simulink model "Mdl_Dim"  (R2024b)
settings: Solver=FixedStepDiscrete  StartTime=0.0  StopTime=10.0  FixedStep=0.1  RelTol=1e-3  EnableMultiTasking=on
values from neighbouring files (symbols this model uses):
  DEFAULT_MODE = mpt.Parameter    [Mdl_Dim_DD.m]
  DEFAULT_STEP = mpt.Parameter    [Mdl_Dim_DD.m]
  Mdl_Dim_cTaskPeriod = mpt.Parameter    [Mdl_Dim_rte_types.m]
  RTE_E_MAX_AGE_EXCEEDED = mpt.Parameter    [Mdl_Dim_rte_types.m]
  RTE_E_NEVER_RECEIVED = mpt.Parameter    [Mdl_Dim_rte_types.m]
  STATUS_OFF = mpt.Parameter    [Mdl_Dim_DD.m]
  STATUS_ON = mpt.Parameter    [Mdl_Dim_DD.m]
  SWITCHING_MECHANISM = mpt.Parameter    [Mdl_Dim_DD.m]
  ZERO_VAL = mpt.Parameter    [Mdl_Dim_DD.m]
undefined symbols (not defined in the file or in its folder): AppModule, CAN_COMUN_ACTIVE, CAN_COMUN_FAIL, CAN_VAL_OFF, CAN_VAL_ON, ChannelID, CLUSTER_ACTIVE, DAYNIGHT_STS_NOTRequire, DIAG_NCTRL, DIM_DAY_MODE, DIM_NIGHT_MODE, DOWN_THRESH_1SW, DrvRec_Rheo_down_Long_Press, DrvRec_Rheo_down_Short_Press, DrvRec_Rheo_up_Long_Press, DrvRec_Rheo_Up_Short_Press, DW_EVENT, DW_ON, eAppMdl_type_instance, eDayNightModeIn, eIllumination_levelIn, eSIGNAL_MISSING, eSIGNAL_NEVER_RECEIVED, eSleepSt_type_instance, FALSE, GetPwmDirect, GetPwmWithTime, GetPwmWithTimeExp, IgnOn, INDEX_MCUID0340, INDEX_MCUID0341, INDEX_MCUID0430, IoHwAb_PwmSignalIdType_type_instance, l_Wheel_Down_ParamArray, l_Wheel_Up_ParamArray, MAX_UINT16, MAXHOLD, MINHOLD, NETWORK_NORMAL, NETWORK_SLEEP, NETWORK_STANDALONE, NONE, NVM_Adapter_SetNVM_RheostatDayStep, NVM_Adapter_SetNVM_RheostatDayStepU1, NVM_Adapter_SetNVM_RheostatDayStepU2, NVM_Adapter_SetNVM_RheostatDayStepU3, NVM_Adapter_SetNVM_RheostatNightStep, NVM_Adapter_SetNVM_RheostatNightStepU1, NVM_Adapter_SetNVM_RheostatNightStepU2, NVM_Adapter_SetNVM_RheostatNightStepU3, OpeModeRheostatChange, pJustRcvdStatus, pNvmData, POS_MAX, POS_MIN, RHEO_1SW_TYPE, RHEO_2SW_TYPE, RHEO_SOFTSW_TYPE, RHEO_VALUE_FIVE_U16, RHEO_VALUE_ONE_BOOL ... (+48)
libraries: simulink x65
(part 1 of 4)
settings Model: Creator=AELANGO6  LastModifiedBy=AELANGO6
settings DataIOCC: SaveOutput=off
settings OptimizationCC: DefaultParameterBehavior=Inlined  EnhancedBackFolding=on  PassReuseOutputArgsAs=Individual arguments  ZeroExternalMemoryAtStartup=off  ZeroInternalMemoryAtStartup=off  MaxStackSize=750  OptimizeBlockOrder=speed  DifferentSizesBufferReuse=on  OptimizationCustomize=off  EfficientTunableParamExpr=on
settings DebuggingCC: ParameterTunabilityLossMsg=error
settings SFSimCC: MATLABDynamicMemAlloc=off
settings RTWCC: Description=AUTOSAR  SystemTargetFile=autosar.tlc  GenCodeOnly=on  TemplateMakefile=ert_default_tmf  PortableWordSizes=on  DataTypeReplacement=CDataTypesFixedWidth
settings CodeAppCC: ForceParamTrailComments=on  IgnoreCustomStorageClasses=off  OperatorAnnotations=on  SimulinkDataObjDesc=on  SFDataObjDesc=on  InsertBlockDesc=on
settings STFCustomTargetCC: TargetLangStandard=C99 (ISO)  MultiwordLength=256  ParMdlRefBuildCompliant=on  CompOptLevelCompliant=on  IncludeMdlTerminateFcn=off  CombineOutputUpdateFcns=on  SuppressErrorStatus=on  ERTCustomFileBanners=on  SupportNonFinite=off  SupportComplex=off  SupportContinuousTime=off  SupportNonInlinedSFcns=off  RemoveResetFunc=on  ParenthesesLevel=Maximum  CastingMode=Standards  MATLABClassNameForMDSCustomization=Simulink.SoftwareTarget.ERTCustomization  AutosarCompliant=on  UseToolchainInfoCompliant=on  LookupTableObjectStructAxisOrder=2,1,3,4,...  LUTObjectStructOrderEvenSpacing=Size,Table,Breakpoints  SystemTargetFile=autosar.tlc
settings ERTTargetCC: TargetLangStandard=C99 (ISO)  ConcurrentExecutionCompliant=off  IncludeMdlTerminateFcn=off  SuppressErrorStatus=on  SupportNonFinite=off  SupportComplex=off  ParenthesesLevel=Maximum  CastingMode=Standards  ModelStepFunctionPrototypeControlCompliant=off  CPPClassGenCompliant=off  AutosarCompliant=on  LookupTableObjectStructAxisOrder=2,1,3,4,...  LUTObjectStructOrderEvenSpacing=Size,Table,Breakpoints  ERTCustomFileTemplate=example_file_process.tlc  ERTFilePackagingFormat=CompactWithDataFile  BooleanTrueId=TRUE  BooleanFalseId=FALSE

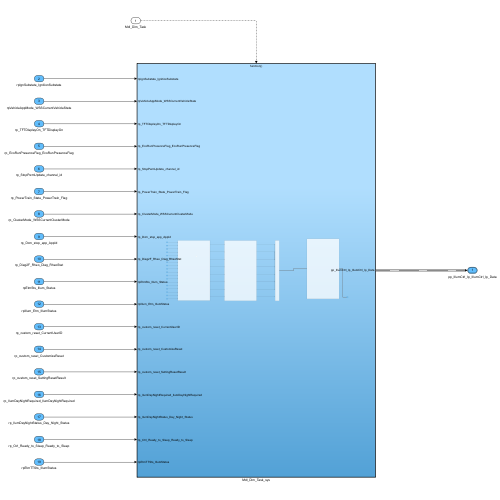
[thumbnail: Simulink's stored preview of the top-level diagram]
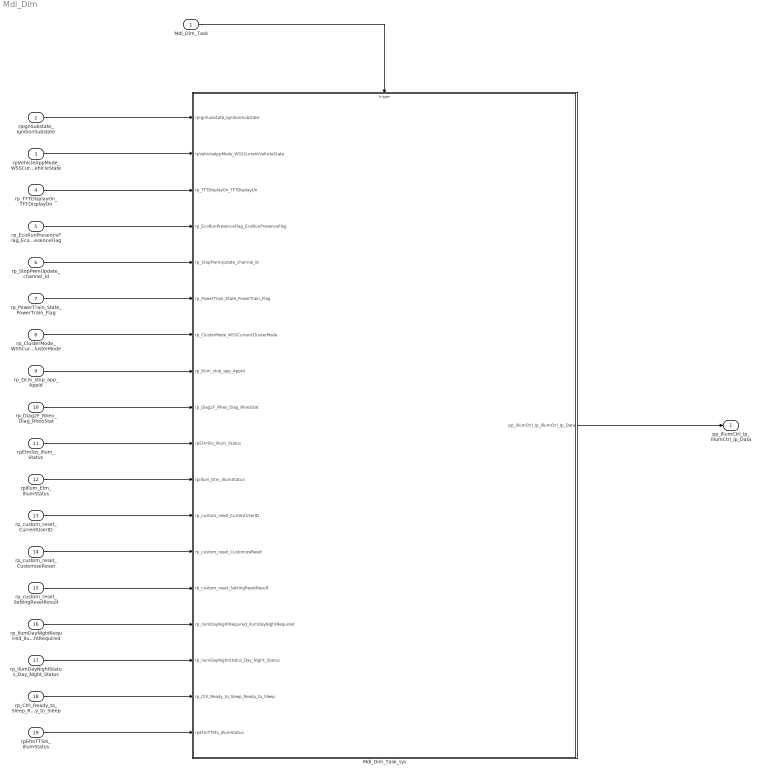
== system Mdl_Dim ==
  Mdl_Dim_Task : Inport  SampleTime=0.1  OutputFunctionCall=on
  rpIgnSubstate_IgnitionSubstate : Inport  Port=2  OutDataTypeStr=IgntionSubstateType  PortDimensions=1
  rpVehicleAppMode_WSSCurrentVehicleState : Inport  Port=3  OutDataTypeStr=VehicleActiveModes  PortDimensions=1
  rp_TFTDisplayOn_TFTDisplayOn : Inport  Port=4  OutDataTypeStr=DisplayStatus  PortDimensions=1
  rp_EcoRunPresenceFlag_EcoRunPresenceFlag : Inport  Port=5  OutDataTypeStr=uint8  PortDimensions=1
  rp_StopPwmUpdate_channel_id : Inport  Port=6  OutDataTypeStr=uint8  PortDimensions=1
  rp_PowerTrain_State_PowerTrain_Flag : Inport  Port=7  OutDataTypeStr=uint8  PortDimensions=1
  rp_ClusterMode_WSSCurrentClusterMode : Inport  Port=8  OutDataTypeStr=ClusterModes  PortDimensions=1
  rp_Dcm_stop_app_AppId : Inport  Port=9  OutDataTypeStr=IOCtrl_Type  PortDimensions=1
  rp_Diag2F_Rheo_Diag_RheoStat : Inport  Port=10  OutDataTypeStr=uint8  PortDimensions=1
  rpEtmSts_Illum_Status : Inport  Port=11  OutDataTypeStr=uint8  PortDimensions=1
  rpIllum_Etm_IllumStatus : Inport  Port=12  OutDataTypeStr=uint8  PortDimensions=1
  rp_custom_reset_CurrentUserID : Inport  Port=13  OutDataTypeStr=UserIdType  PortDimensions=1
  rp_custom_reset_CustomizeReset : Inport  Port=14  OutDataTypeStr=CustResetType  PortDimensions=1
  rp_custom_reset_SettingResetResult : Inport  Port=15  OutDataTypeStr=SettingResetResult_Type  PortDimensions=1
  rp_IlumDayNightRequired_IlumDayNightRequired : Inport  Port=16  OutDataTypeStr=uint8  PortDimensions=1
  rp_IlumDayNightStatus_Day_Night_Status : Inport  Port=17  OutDataTypeStr=uint8  PortDimensions=1
  rp_Ctrl_Ready_to_Sleep_Ready_to_Sleep : Inport  Port=18  OutDataTypeStr=boolean  PortDimensions=1
  rpEtmTTSts_IllumStatus : Inport  Port=19  OutDataTypeStr=uint8  PortDimensions=1
  Mdl_Dim_Task_sys : Subsystem  TreatAsAtomicUnit=on
  pp_IllumCtrl_Ip_IllumCtrl_Ip_Data : Outport  OutDataTypeStr=Bus:IllumCtrl_Ip
  wires:
  Mdl_Dim_Task/1 -> Mdl_Dim_Task_sys/Trigger
  rp_PowerTrain_State_PowerTrain_Flag/1 -> Mdl_Dim_Task_sys/6(rp_PowerTrain_State_PowerTrain_Flag)
  rpIgnSubstate_IgnitionSubstate/1 -> Mdl_Dim_Task_sys/1(rpIgnSubstate_IgnitionSubstate)
  rp_custom_reset_CurrentUserID/1 -> Mdl_Dim_Task_sys/12(rp_custom_reset_CurrentUserID)
  rpVehicleAppMode_WSSCurrentVehicleState/1 -> Mdl_Dim_Task_sys/2(rpVehicleAppMode_WSSCurrentVehicleState)
  rp_TFTDisplayOn_TFTDisplayOn/1 -> Mdl_Dim_Task_sys/3(rp_TFTDisplayOn_TFTDisplayOn)
  rp_IlumDayNightStatus_Day_Night_Status/1 -> Mdl_Dim_Task_sys/16(rp_IlumDayNightStatus_Day_Night_Status)
  rp_EcoRunPresenceFlag_EcoRunPresenceFlag/1 -> Mdl_Dim_Task_sys/4(rp_EcoRunPresenceFlag_EcoRunPresenceFlag)
  rp_StopPwmUpdate_channel_id/1 -> Mdl_Dim_Task_sys/5(rp_StopPwmUpdate_channel_id)
  rp_ClusterMode_WSSCurrentClusterMode/1 -> Mdl_Dim_Task_sys/7(rp_ClusterMode_WSSCurrentClusterMode)
  rp_Dcm_stop_app_AppId/1 -> Mdl_Dim_Task_sys/8(rp_Dcm_stop_app_AppId)
  rp_Diag2F_Rheo_Diag_RheoStat/1 -> Mdl_Dim_Task_sys/9(rp_Diag2F_Rheo_Diag_RheoStat)
  rpEtmSts_Illum_Status/1 -> Mdl_Dim_Task_sys/10(rpEtmSts_Illum_Status)
  rpIllum_Etm_IllumStatus/1 -> Mdl_Dim_Task_sys/11(rpIllum_Etm_IllumStatus)
  rp_custom_reset_CustomizeReset/1 -> Mdl_Dim_Task_sys/13(rp_custom_reset_CustomizeReset)
  rp_custom_reset_SettingResetResult/1 -> Mdl_Dim_Task_sys/14(rp_custom_reset_SettingResetResult)
  rp_IlumDayNightRequired_IlumDayNightRequired/1 -> Mdl_Dim_Task_sys/15(rp_IlumDayNightRequired_IlumDayNightRequired)
  rp_Ctrl_Ready_to_Sleep_Ready_to_Sleep/1 -> Mdl_Dim_Task_sys/17(rp_Ctrl_Ready_to_Sleep_Ready_to_Sleep)
  Mdl_Dim_Task_sys/1(pp_IllumCtrl_Ip_IllumCtrl_Ip_Data) -> pp_IllumCtrl_Ip_IllumCtrl_Ip_Data/1
  rpEtmTTSts_IllumStatus/1 -> Mdl_Dim_Task_sys/18(rpEtmTTSts_IllumStatus)

== system Mdl_Dim/Mdl_Dim_Task_sys ==
  rpIgnSubstate_IgnitionSubstate : Inport  OutDataTypeStr=IgntionSubstateType  PortDimensions=1
  rpVehicleAppMode_WSSCurrentVehicleState : Inport  Port=2  OutDataTypeStr=VehicleActiveModes  PortDimensions=1
  rp_TFTDisplayOn_TFTDisplayOn : Inport  Port=3  OutDataTypeStr=DisplayStatus  PortDimensions=1
  rp_EcoRunPresenceFlag_EcoRunPresenceFlag : Inport  Port=4  OutDataTypeStr=uint8  PortDimensions=1
  rp_StopPwmUpdate_channel_id : Inport  Port=5  OutDataTypeStr=uint8  PortDimensions=1
  rp_PowerTrain_State_PowerTrain_Flag : Inport  Port=6  OutDataTypeStr=uint8  PortDimensions=1
  rp_ClusterMode_WSSCurrentClusterMode : Inport  Port=7  OutDataTypeStr=ClusterModes  PortDimensions=1
  rp_Dcm_stop_app_AppId : Inport  Port=8  OutDataTypeStr=IOCtrl_Type  PortDimensions=1
  rp_Diag2F_Rheo_Diag_RheoStat : Inport  Port=9  OutDataTypeStr=uint8  PortDimensions=1
  rpEtmSts_Illum_Status : Inport  Port=10  OutDataTypeStr=uint8  PortDimensions=1
  rpIllum_Etm_IllumStatus : Inport  Port=11  OutDataTypeStr=uint8  PortDimensions=1
  rp_custom_reset_CurrentUserID : Inport  Port=12  OutDataTypeStr=UserIdType  PortDimensions=1
  rp_custom_reset_CustomizeReset : Inport  Port=13  OutDataTypeStr=CustResetType  PortDimensions=1
  rp_custom_reset_SettingResetResult : Inport  Port=14  OutDataTypeStr=SettingResetResult_Type  PortDimensions=1
  rp_IlumDayNightRequired_IlumDayNightRequired : Inport  Port=15  OutDataTypeStr=uint8  PortDimensions=1
  rp_IlumDayNightStatus_Day_Night_Status : Inport  Port=16  OutDataTypeStr=uint8  PortDimensions=1
  rp_Ctrl_Ready_to_Sleep_Ready_to_Sleep : Inport  Port=17  OutDataTypeStr=boolean  PortDimensions=1
  rpEtmTTSts_IllumStatus : Inport  Port=18  OutDataTypeStr=uint8  PortDimensions=1
  function : TriggerPort  TriggerType=function-call  VariantControl=(inherit)  SampleTimeType=periodic  SampleTime=-1
  IllumCtrl_Ip_Data_creator : BusCreator  Inputs=8  OutDataTypeStr=Bus:IllumCtrl_Ip  NonVirtualBus=on
  InputHarness : Subsystem  Variant=on
  OutputHarness : Subsystem  Variant=on
  Subsystem : Subsystem
  pp_IllumCtrl_Ip_IllumCtrl_Ip_Data : Outport  OutDataTypeStr=Bus:IllumCtrl_Ip  PortDimensions=1
  wires:
  rpIgnSubstate_IgnitionSubstate/1 -> InputHarness/1(rpIgnSubstate_IgnitionSubstate)
  rpVehicleAppMode_WSSCurrentVehicleState/1 -> InputHarness/2(rpVehicleAppMode_WSSCurrentVehicleState)
  rp_TFTDisplayOn_TFTDisplayOn/1 -> InputHarness/3(rp_TFTDisplayOn_TFTDisplayOn)
  rp_EcoRunPresenceFlag_EcoRunPresenceFlag/1 -> InputHarness/4(rp_EcoRunPresenceFlag_EcoRunPresenceFlag)
  rp_StopPwmUpdate_channel_id/1 -> InputHarness/5(rp_StopPwmUpdate_channel_id)
  rp_PowerTrain_State_PowerTrain_Flag/1 -> InputHarness/6(rp_PowerTrain_State_PowerTrain_Flag)
  rp_ClusterMode_WSSCurrentClusterMode/1 -> InputHarness/7(rp_ClusterMode_WSSCurrentClusterMode)
  rp_Dcm_stop_app_AppId/1 -> InputHarness/8(rp_Dcm_stop_app_AppId)
  rp_Diag2F_Rheo_Diag_RheoStat/1 -> InputHarness/9(rp_Diag2F_Rheo_Diag_RheoStat)
  rpEtmSts_Illum_Status/1 -> InputHarness/10(rpEtmSts_Illum_Status)
  rpIllum_Etm_IllumStatus/1 -> InputHarness/11(rpIllum_Etm_IllumStatus)
  rp_custom_reset_CurrentUserID/1 -> InputHarness/12(rp_custom_reset_CurrentUserID)
  rp_custom_reset_CustomizeReset/1 -> InputHarness/13(rp_custom_reset_CustomizeReset)
  rp_custom_reset_SettingResetResult/1 -> InputHarness/14(rp_custom_reset_SettingResetResult)
  rp_IlumDayNightRequired_IlumDayNightRequired/1 -> InputHarness/15(rp_IlumDayNightRequired_IlumDayNightRequired)
  rp_IlumDayNightStatus_Day_Night_Status/1 -> InputHarness/16(rp_IlumDayNightStatus_Day_Night_Status)
  rp_Ctrl_Ready_to_Sleep_Ready_to_Sleep/1 -> InputHarness/17(rp_Ctrl_Ready_to_Sleep_Ready_to_Sleep)
  rpEtmTTSts_IllumStatus/1 -> InputHarness/18(rpEtmTTSts_IllumStatus)
  InputHarness/1(rpIgnSubstate_IgnitionSubstate_out) -> Subsystem/1(IgnitionSubstate)
  InputHarness/2(rpVehicleAppMode_WSSCurrentVehicleState_out) -> Subsystem/2(VehicleState)
  InputHarness/3(rp_TFTDisplayOn_TFTDisplayOn_out) -> Subsystem/3(TFTDisplayOn)
  InputHarness/4(rp_ClusterMode_WSSCurrentClusterMode_out) -> Subsystem/4(cluster_Active_check)
  OutputHarness/1(pp_IllumCtrl_Ip_IllumCtrl_Ip_Data) -> pp_IllumCtrl_Ip_IllumCtrl_Ip_Data/1
  IllumCtrl_Ip_Data_creator/1 -> OutputHarness/1(pp_IllumCtrl_Ip_IllumCtrl_Ip_Data_in)  "fl_IllumMdl_Op"
  InputHarness/5(IL_Mode_CAN_Data) -> Subsystem/5(IL_Mode_Can_Data)
  InputHarness/6(IL_Mode_CAN_Status) -> Subsystem/6(IL_Mode_Can_Sts)
  InputHarness/7(IL_Level_CAN_Data) -> Subsystem/7(IL_Level_Can_Data)
  InputHarness/8(IL_Level_CAN_Status) -> Subsystem/8(IL_Level_Can_Sts)
  Subsystem/1(power_mode) -> IllumCtrl_Ip_Data_creator/4  "power_mode"
  Subsystem/2(Illumination_Sts) -> IllumCtrl_Ip_Data_creator/3  "Illumination_Sts"
  Subsystem/3(Illumination_Mode) -> IllumCtrl_Ip_Data_creator/1  "Illumination_Mode"
  Subsystem/4(step_value) -> IllumCtrl_Ip_Data_creator/5  "step_value"
  Subsystem/5(switch_type) -> IllumCtrl_Ip_Data_creator/7  "switch_type"
  Subsystem/6(battery_status) -> IllumCtrl_Ip_Data_creator/2  "battery_status"
  Subsystem/7(step_direction) -> IllumCtrl_Ip_Data_creator/6  "step_direction"
  Subsystem/8(derating_value) -> IllumCtrl_Ip_Data_creator/8  "Derating_Value"

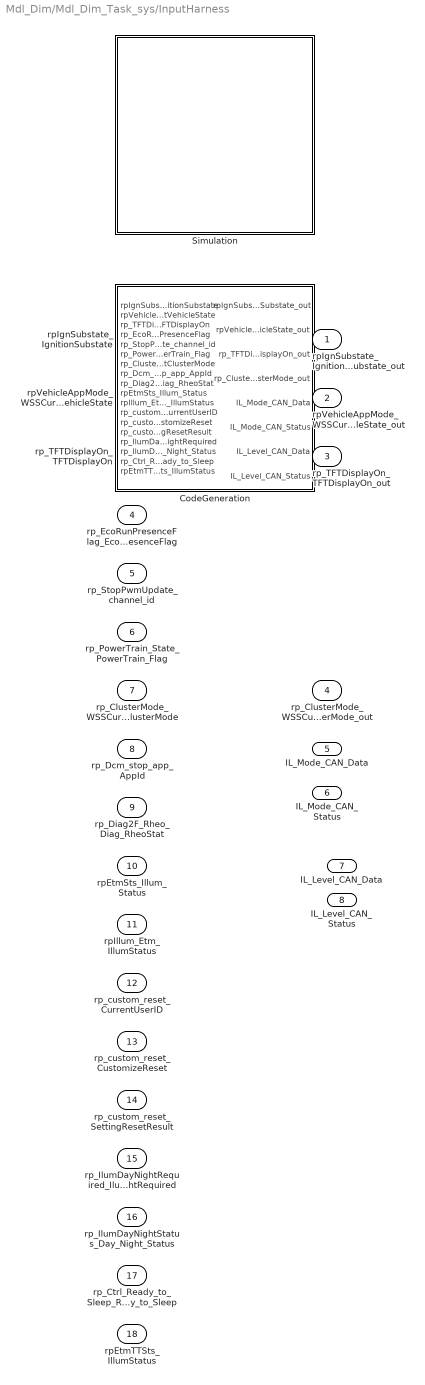
== system Mdl_Dim/Mdl_Dim_Task_sys/InputHarness ==
  rpIgnSubstate_IgnitionSubstate : Inport  OutDataTypeStr=IgntionSubstateType  PortDimensions=1
  rpVehicleAppMode_WSSCurrentVehicleState : Inport  Port=2  OutDataTypeStr=VehicleActiveModes  PortDimensions=1
  rp_TFTDisplayOn_TFTDisplayOn : Inport  Port=3  OutDataTypeStr=DisplayStatus  PortDimensions=1
  rp_EcoRunPresenceFlag_EcoRunPresenceFlag : Inport  Port=4  OutDataTypeStr=uint8  PortDimensions=1
  rp_StopPwmUpdate_channel_id : Inport  Port=5  OutDataTypeStr=uint8  PortDimensions=1
  rp_PowerTrain_State_PowerTrain_Flag : Inport  Port=6  OutDataTypeStr=uint8  PortDimensions=1
  rp_ClusterMode_WSSCurrentClusterMode : Inport  Port=7  OutDataTypeStr=ClusterModes  PortDimensions=1
  rp_Dcm_stop_app_AppId : Inport  Port=8  OutDataTypeStr=IOCtrl_Type  PortDimensions=1
  rp_Diag2F_Rheo_Diag_RheoStat : Inport  Port=9  OutDataTypeStr=uint8  PortDimensions=1
  rpEtmSts_Illum_Status : Inport  Port=10  OutDataTypeStr=uint8  PortDimensions=1
  rpIllum_Etm_IllumStatus : Inport  Port=11  OutDataTypeStr=uint8  PortDimensions=1
  rp_custom_reset_CurrentUserID : Inport  Port=12  OutDataTypeStr=UserIdType  PortDimensions=1
  rp_custom_reset_CustomizeReset : Inport  Port=13  OutDataTypeStr=CustResetType  PortDimensions=1
  rp_custom_reset_SettingResetResult : Inport  Port=14  OutDataTypeStr=SettingResetResult_Type  PortDimensions=1
  rp_IlumDayNightRequired_IlumDayNightRequired : Inport  Port=15  OutDataTypeStr=uint8  PortDimensions=1
  rp_IlumDayNightStatus_Day_Night_Status : Inport  Port=16  OutDataTypeStr=uint8  PortDimensions=1
  rp_Ctrl_Ready_to_Sleep_Ready_to_Sleep : Inport  Port=17  OutDataTypeStr=boolean  PortDimensions=1
  rpEtmTTSts_IllumStatus : Inport  Port=18  OutDataTypeStr=uint8  PortDimensions=1
  CodeGeneration : Subsystem  VariantControl=CODEGENERATION
  Simulation : Subsystem  VariantControl=SIMULATION
  rpIgnSubstate_IgnitionSubstate_out : Outport  OutDataTypeStr=IgntionSubstateType  PortDimensions=1
  rpVehicleAppMode_WSSCurrentVehicleState_out : Outport  Port=2  OutDataTypeStr=VehicleActiveModes  PortDimensions=1
  rp_TFTDisplayOn_TFTDisplayOn_out : Outport  Port=3  OutDataTypeStr=DisplayStatus  PortDimensions=1
  rp_ClusterMode_WSSCurrentClusterMode_out : Outport  Port=4  OutDataTypeStr=ClusterModes  PortDimensions=1
  IL_Mode_CAN_Data : Outport  Port=5
  IL_Mode_CAN_Status : Outport  Port=6
  IL_Level_CAN_Data : Outport  Port=7
  IL_Level_CAN_Status : Outport  Port=8

== system Mdl_Dim/Mdl_Dim_Task_sys/OutputHarness ==
  pp_IllumCtrl_Ip_IllumCtrl_Ip_Data_in : Inport  OutDataTypeStr=Bus:IllumCtrl_Ip  PortDimensions=1
  CodeGeneration : Subsystem  VariantControl=CODEGENERATION
  Simulation : Subsystem  VariantControl=SIMULATION
  pp_IllumCtrl_Ip_IllumCtrl_Ip_Data : Outport  OutDataTypeStr=Bus:IllumCtrl_Ip  PortDimensions=1

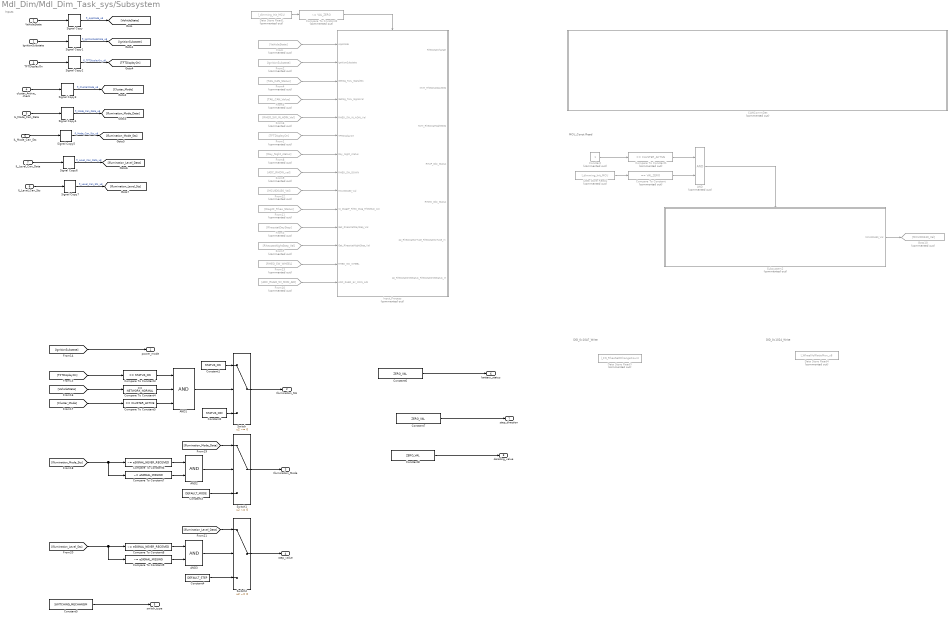
== system Mdl_Dim/Mdl_Dim_Task_sys/Subsystem ==
  note: Inputs
  note: MCU_Const Read
  note: DID_0x10A7_Write
  note: DID_0x1024_Write
  IgnitionSubstate : Inport
  VehicleState : Inport  Port=2
  TFTDisplayOn : Inport  Port=3
  cluster_Active_check : Inport  Port=4
  IL_Mode_Can_Data : Inport  Port=5
  IL_Mode_Can_Sts : Inport  Port=6
  IL_Level_Can_Data : Inport  Port=7
  IL_Level_Can_Sts : Inport  Port=8
  AND : Logic  Commented=on  AllPortsSameDT=off  OutDataTypeStr=boolean
  AND1 : Logic  Inputs=3  AllPortsSameDT=off  OutDataTypeStr=boolean
  AND2 : Logic  AllPortsSameDT=off  OutDataTypeStr=boolean
  AND3 : Logic  AllPortsSameDT=off  OutDataTypeStr=boolean
  CANCommDet : Subsystem  Commented=on  TreatAsAtomicUnit=on
  Compare To Constant : simulink/Logic and Bit Operations/Compare To Constant  Commented=on  relop===  const=VAL_ZERO  OutDataTypeStr=boolean
  Compare To Constant1 : simulink/Logic and Bit Operations/Compare To Constant  Commented=on  relop===  const=CLUSTER_ACTIVE  OutDataTypeStr=boolean
  Compare To Constant2 : simulink/Logic and Bit Operations/Compare To Constant  Commented=on  relop=~=  const=VAL_ZERO  OutDataTypeStr=boolean
  Compare To Constant3 : simulink/Logic and Bit Operations/Compare To Constant  relop===  const=STATUS_ON  OutDataTypeStr=boolean
  Compare To Constant4 : simulink/Logic and Bit Operations/Compare To Constant  relop===  const=NETWORK_NORMAL  OutDataTypeStr=boolean
  Compare To Constant5 : simulink/Logic and Bit Operations/Compare To Constant  relop===  const=CLUSTER_ACTIVE  OutDataTypeStr=boolean
  Compare To Constant6 : simulink/Logic and Bit Operations/Compare To Constant  relop=~=  const=eSIGNAL_NEVER_RECEIVED  OutDataTypeStr=boolean
  Compare To Constant7 : simulink/Logic and Bit Operations/Compare To Constant  relop=~=  const=eSIGNAL_MISSING  OutDataTypeStr=boolean
  Compare To Constant8 : simulink/Logic and Bit Operations/Compare To Constant  relop=~=  const=eSIGNAL_NEVER_RECEIVED  OutDataTypeStr=boolean
  Compare To Constant9 : simulink/Logic and Bit Operations/Compare To Constant  relop=~=  const=eSIGNAL_MISSING  OutDataTypeStr=boolean
  Constant : Constant  Commented=on
  Constant1 : Constant  Value=STATUS_ON
  Constant2 : Constant  Value=STATUS_OFF
  Constant3 : Constant  Value=DEFAULT_MODE
  Constant4 : Constant  Value=DEFAULT_STEP
  Constant5 : Constant  Value=SWITCHING_MECHANISM
  Constant6 : Constant  Value=ZERO_VAL
  Constant7 : Constant  Value=ZERO_VAL
  Constant8 : Constant  Value=ZERO_VAL
  Data Store Read1 : DataStoreRead  Commented=on  DataStoreName=l_dimming_Init_MCU  IndexOptions=Index vector (dialog)  Indices=1  OutputSizes=1
  Data Store Read2 : DataStoreRead  Commented=on  DataStoreName=l_dimming_Init_MCU  IndexOptions=Index vector (dialog)  Indices=1  OutputSizes=1
  Data Store Read3 : DataStoreRead  Commented=on  DataStoreName=l_FN_RheoSettChangeCount  IndexOptions=Index vector (dialog)  Indices=1  OutputSizes=1
  Data Store Read4 : DataStoreRead  Commented=on  DataStoreName=l_WheelVolRatioMon_u8  IndexOptions=Index vector (dialog)  Indices=1  OutputSizes=1
  From : From  Commented=on  GotoTag=VehicleState
  From1 : From  Commented=on  GotoTag=TFTDisplayOn
  From10 : From  Commented=on  GotoTag=ADC_RHEO_5V_MON_ADI
  From11 : From  Commented=on  GotoTag=Diag2F_Rheo_Status
  From12 : From  Commented=on  GotoTag=MCUID0430_Val
  From13 : From  Commented=on  GotoTag=RHEO_SW_WHEEL
  From2 : From  Commented=on  GotoTag=IgnitionSubstate
  From3 : From  Commented=on  GotoTag=RheostatDayStep
  From4 : From  Commented=on  GotoTag=TAIL_CAN_Status
  From5 : From  Commented=on  GotoTag=TAIL_CAN_Value
  From6 : From  Commented=on  GotoTag=RHEO_SW_IN_ADIN_Val
  From7 : From  Commented=on  GotoTag=RheostatNightStep_Val
  From8 : From  Commented=on  GotoTag=Day_Night_status
  From9 : From  Commented=on  GotoTag=ADC_RHDW_val
  Goto10 : Goto  Commented=on  GotoTag=MCUID0430_Val
  Input_Process : Subsystem  Priority=1  Commented=on  RTWFcnName=fl_input_Process
      settings: RTWSystemCode=Nonreusable function  RTWFcnNameOpts=User specified
  Signal Copy{,1..7} (8 alike) : SignalConversion  OverrideOpt=off
  Subsystem2 : Subsystem  Commented=on  RTWFcnName=MCUConst_Read
      settings: RTWSystemCode=Nonreusable function  RTWFcnNameOpts=User specified  FunctionInterfaceSpec=Allow arguments (Optimized)
  Switch : Switch  Criteria=u2 ~= 0  SaturateOnIntegerOverflow=off  InputSameDT=off
  Switch1 : Switch  Criteria=u2 ~= 0  SaturateOnIntegerOverflow=off  InputSameDT=off
  Switch2 : Switch  Criteria=u2 ~= 0  SaturateOnIntegerOverflow=off  InputSameDT=off
  power_mode : Outport
  Illumination_Sts : Outport  Port=2
  Illumination_Mode : Outport  Port=3
  step_value : Outport  Port=4
  switch_type : Outport  Port=5
  battery_status : Outport  Port=6
  step_direction : Outport  Port=7
  derating_value : Outport  Port=8
  wires:
  From/1 -> Input_Process/1(AppMode)
  From2/1 -> Input_Process/2(IgnitionSubstate)
  VehicleState/1 -> Signal Copy/1
  IgnitionSubstate/1 -> Signal Copy1/1
  TFTDisplayOn/1 -> Signal Copy2/1
  From1/1 -> Input_Process/6(TFTDisplayOn)
  Signal Copy/1 -> [VehicleState]  "fl_AppMode_u8"
  Signal Copy1/1 -> [IgnitionSubstate]  "fl_IgnitionSubstate_u8"
  Signal Copy2/1 -> [TFTDisplayOn]  "fl_TFTDisplayOn_u8"
  From3/1 -> Input_Process/11(Get_RheostatDayStep_Val)
  From4/1 -> Input_Process/3(GetSig_TAIL_SignalSts)
  From5/1 -> Input_Process/4(GetSig_TAIL_SignalVal)
  From6/1 -> Input_Process/5(RHEO_SW_IN_ADIN_Val)
  From7/1 -> Input_Process/12(Get_RheostatNightStep_Val)
  From8/1 -> Input_Process/7(Day_Night_status)
  From9/1 -> Input_Process/8(RHEO_SW_DOWN)
  From12/1 -> Input_Process/9(MCUID0430_Val)
  From11/1 -> Input_Process/10(rp_Diag2F_Rheo_Diag_RheoStat_out)
  From10/1 -> Input_Process/14(ADC_RHEO_5V_MON_ADI)
  From13/1 -> Input_Process/13(RHEO_SW_WHEEL)
  Data Store Read2/1 -> Compare To Constant/1
  Constant/1 -> Compare To Constant1/1
  Compare To Constant/1 -> AND/2
  Compare To Constant1/1 -> AND/1
  AND/1 -> Subsystem2/Enable
  Subsystem2/1(MCUID0430_Val) -> Goto10/1
  Data Store Read1/1 -> Compare To Constant2/1
  Compare To Constant2/1 -> Input_Process/Enable
  cluster_Active_check/1 -> Signal Copy3/1
  Signal Copy3/1 -> [Cluster_Mode]  "fl_ClusterMode_u8"
  IL_Mode_Can_Data/1 -> Signal Copy4/1
  Signal Copy4/1 -> [Illumination_Mode_Data]  "fl_Mode_Can_Data_u8"
  IL_Mode_Can_Sts/1 -> Signal Copy5/1
  Signal Copy5/1 -> [Illumination_Mode_Sts]  "fl_Mode_Can_Sts_u8"
  IL_Level_Can_Data/1 -> Signal Copy6/1
  Signal Copy6/1 -> [Illumination_Level_Data]  "fl_Level_Can_Data_u8"
  IL_Level_Can_Sts/1 -> Signal Copy7/1
  Signal Copy7/1 -> [Illumination_Level_Sts]  "fl_Level_Can_Sts_u8"
  [IgnitionSubstate] -> power_mode/1
  [TFTDisplayOn] -> Compare To Constant3/1
  [Cluster_Mode] -> Compare To Constant5/1
  [VehicleState] -> Compare To Constant4/1
  Compare To Constant5/1 -> AND1/3
  Compare To Constant4/1 -> AND1/2
  Compare To Constant3/1 -> AND1/1
  AND1/1 -> Switch/2
  Constant1/1 -> Switch/1
  Constant2/1 -> Switch/3
  Switch/1 -> Illumination_Sts/1
  [Illumination_Mode_Sts] -> Compare To Constant7/1, Compare To Constant6/1
  Compare To Constant6/1 -> AND2/1
  Compare To Constant7/1 -> AND2/2
  AND2/1 -> Switch1/2
  [Illumination_Mode_Data] -> Switch1/1
  Constant3/1 -> Switch1/3
  Switch1/1 -> Illumination_Mode/1
  AND3/1 -> Switch2/2
  Constant4/1 -> Switch2/3
  Switch2/1 -> step_value/1
  [Illumination_Level_Data] -> Switch2/1
  Compare To Constant9/1 -> AND3/2
  Compare To Constant8/1 -> AND3/1
  [Illumination_Level_Sts] -> Compare To Constant9/1, Compare To Constant8/1
  Constant5/1 -> switch_type/1
  Constant6/1 -> battery_status/1
  Constant7/1 -> step_direction/1
  Constant8/1 -> derating_value/1

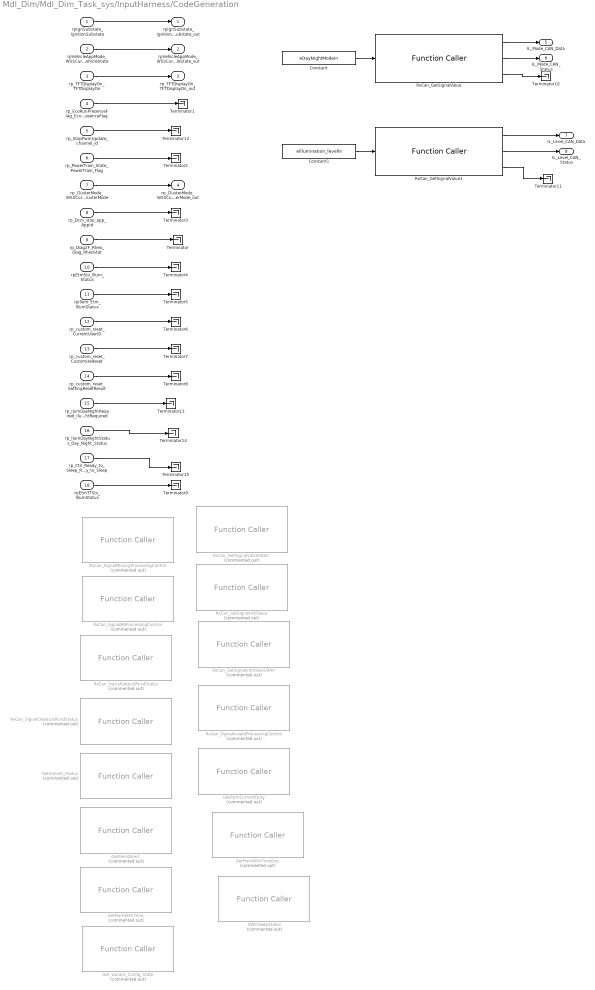
== system Mdl_Dim/Mdl_Dim_Task_sys/InputHarness/CodeGeneration ==
  rpIgnSubstate_IgnitionSubstate : Inport  OutDataTypeStr=IgntionSubstateType  PortDimensions=1
  rpVehicleAppMode_WSSCurrentVehicleState : Inport  Port=2  OutDataTypeStr=VehicleActiveModes  PortDimensions=1
  rp_TFTDisplayOn_TFTDisplayOn : Inport  Port=3  OutDataTypeStr=DisplayStatus  PortDimensions=1
  rp_EcoRunPresenceFlag_EcoRunPresenceFlag : Inport  Port=4  OutDataTypeStr=uint8  PortDimensions=1
  rp_StopPwmUpdate_channel_id : Inport  Port=5  OutDataTypeStr=uint8  PortDimensions=1
  rp_PowerTrain_State_PowerTrain_Flag : Inport  Port=6  OutDataTypeStr=uint8  PortDimensions=1
  rp_ClusterMode_WSSCurrentClusterMode : Inport  Port=7  OutDataTypeStr=ClusterModes  PortDimensions=1
  rp_Dcm_stop_app_AppId : Inport  Port=8  OutDataTypeStr=IOCtrl_Type  PortDimensions=1
  rp_Diag2F_Rheo_Diag_RheoStat : Inport  Port=9  OutDataTypeStr=uint8  PortDimensions=1
  rpEtmSts_Illum_Status : Inport  Port=10  OutDataTypeStr=uint8  PortDimensions=1
  rpIllum_Etm_IllumStatus : Inport  Port=11  OutDataTypeStr=uint8  PortDimensions=1
  rp_custom_reset_CurrentUserID : Inport  Port=12  OutDataTypeStr=UserIdType  PortDimensions=1
  rp_custom_reset_CustomizeReset : Inport  Port=13  OutDataTypeStr=CustResetType  PortDimensions=1
  rp_custom_reset_SettingResetResult : Inport  Port=14  OutDataTypeStr=SettingResetResult_Type  PortDimensions=1
  rp_IlumDayNightRequired_IlumDayNightRequired : Inport  Port=15  OutDataTypeStr=uint8  PortDimensions=1
  rp_IlumDayNightStatus_Day_Night_Status : Inport  Port=16  OutDataTypeStr=uint8  PortDimensions=1
  rp_Ctrl_Ready_to_Sleep_Ready_to_Sleep : Inport  Port=17  OutDataTypeStr=boolean  PortDimensions=1
  rpEtmTTSts_IllumStatus : Inport  Port=18  OutDataTypeStr=uint8  PortDimensions=1
  Constant : Constant  Value=eDayNightModeIn
  Constant1 : Constant  Value=eIllumination_levelIn
  GetPwmCurrentDuty : FunctionCaller  Commented=on  FunctionPrototype=Channel_Duty = GetPwmCurrentDuty(ChannelID)  InputArgumentSpecifications=uint8(1)  OutputArgumentSpecifications=uint16(1)
  GetPwmDirect : FunctionCaller  Commented=on  FunctionPrototype=GetPwmDirect(ChannelID,TargetDuty)  InputArgumentSpecifications=IoHwAb_PwmSignalIdType_type_instance(1) ,uint16(1)  OutputArgumentSpecifications=<Enter example>
  GetPwmWithTime : FunctionCaller  Commented=on  FunctionPrototype=GetPwmWithTime(ChannelID,TargetDuty,TargetTime)  InputArgumentSpecifications=IoHwAb_PwmSignalIdType_type_instance(1) ,uint16(1) ,uint16(1)  OutputArgumentSpecifications=<Enter example>
  GetPwmWithTimeExp : FunctionCaller  Commented=on  FunctionPrototype=GetPwmWithTimeExp(ChannelID,TargetDuty,TargetTime)  InputArgumentSpecifications=IoHwAb_PwmSignalIdType_type_instance(1) ,uint16(1) ,uint16(1)  OutputArgumentSpecifications=<Enter example>
  GetVariant_Status : FunctionCaller  Commented=on  FunctionPrototype=Variant_Status = GetVariant_Status(Variant_Ind)  InputArgumentSpecifications=uint8(1)  OutputArgumentSpecifications=uint8(1)
  Get_Variant_Config_State : FunctionCaller  Commented=on  FunctionPrototype=VariantActiveSt = Get_Variant_Config_State(VariantID)  InputArgumentSpecifications=uint8(1)  OutputArgumentSpecifications=uint8(1)
  RxCan_GetSignalValue : FunctionCaller  FunctionPrototype=[pSignalValue,pSignalStatus,error_status] = RxCan_GetSignalValue(SignalId)  InputArgumentSpecifications=tRxSignalId_type_instance(1)  OutputArgumentSpecifications=uint8(1) ,tRxSignalStatus_type_instance(1) ,uint8(1)
  RxCan_GetSignalValue1 : FunctionCaller  FunctionPrototype=[pSignalValue,pSignalStatus,error_status] = RxCan_GetSignalValue(SignalId)  InputArgumentSpecifications=tRxSignalId_type_instance(1)  OutputArgumentSpecifications=uint8(1) ,tRxSignalStatus_type_instance(1) ,uint8(1)
  RxCan_GetSignalValueU8Arr : FunctionCaller  Commented=on  FunctionPrototype=[pSignalValue,pSignalStatus,pSignalLength,error_status] = RxCan_GetSignalValueU8Arr(SignalId)  InputArgumentSpecifications=tRxSignalId_type_instance(1)  OutputArgumentSpecifications=uint8(1) ,tRxSignalStatus_type_instance(1) ,uint32(1) ,uint8(1)
  RxCan_SetSignalInitValue : FunctionCaller  Commented=on  FunctionPrototype=[pSignalValue,error_status] = RxCan_SetSignalInitValue(SignalId)  InputArgumentSpecifications=tRxSignalId_type_instance(1)  OutputArgumentSpecifications=uint8(1) ,uint8(1)
  RxCan_SetSignalInitValueU8Arr : FunctionCaller  Commented=on  FunctionPrototype=[pSignaValue,pSignalLength,error_status] = RxCan_SetSignalInitValueU8Arr(SignalId)  InputArgumentSpecifications=tRxSignalId_type_instance(1)  OutputArgumentSpecifications=uint8(1) ,uint32(1) ,uint8(1)
  RxCan_SignalClearJustRcvdStatus : FunctionCaller  Commented=on  FunctionPrototype=RxCan_SignalClearJustRcvdStatus(SignalId)  InputArgumentSpecifications=tRxSignalId_type_instance(1)  OutputArgumentSpecifications=<Enter example>
  RxCan_SignalGetJustRcvdStatus : FunctionCaller  Commented=on  FunctionPrototype=RxCan_SignalGetJustRcvdStatus(SignalId,pJustRcvdStatus)  InputArgumentSpecifications=tRxSignalId_type_instance(1) ,tRxSignalJustRcvdStatus_type_instance(1)  OutputArgumentSpecifications=<Enter example>
  RxCan_SignalInvalidProcessingControl : FunctionCaller  Commented=on  FunctionPrototype=RxCan_SignalInvalidProcessingControl(SignalId,Status)  InputArgumentSpecifications=tRxSignalId_type_instance(1) ,boolean(1)  OutputArgumentSpecifications=<Enter example>
  RxCan_SignalMissingProcessingControl : FunctionCaller  Commented=on  FunctionPrototype=RxCan_SignalMissingProcessingControl(SignalId,Status)  InputArgumentSpecifications=tRxSignalId_type_instance(1) ,boolean(1)  OutputArgumentSpecifications=<Enter example>
  RxCan_SignalNRProcessingControl : FunctionCaller  Commented=on  FunctionPrototype=RxCan_SignalNRProcessingControl(SignalId,Status)  InputArgumentSpecifications=tRxSignalId_type_instance(1) ,boolean(1)  OutputArgumentSpecifications=<Enter example>
  SWCSleepStatus : FunctionCaller  Commented=on  FunctionPrototype=SWCSleepStatus(AppModule,SleepStatus)  InputArgumentSpecifications=eAppMdl_type_instance(1) ,eSleepSt_type_instance(1)  OutputArgumentSpecifications=<Enter example>
  Terminator{,1..15} (16 alike) : Terminator
  rpIgnSubstate_IgnitionSubstate_out : Outport  OutDataTypeStr=IgntionSubstateType  PortDimensions=1
  rpVehicleAppMode_WSSCurrentVehicleState_out : Outport  Port=2  OutDataTypeStr=VehicleActiveModes  PortDimensions=1
  rp_TFTDisplayOn_TFTDisplayOn_out : Outport  Port=3  OutDataTypeStr=DisplayStatus  PortDimensions=1
  rp_ClusterMode_WSSCurrentClusterMode_out : Outport  Port=4  OutDataTypeStr=ClusterModes  PortDimensions=1
  IL_Mode_CAN_Data : Outport  Port=5
  IL_Mode_CAN_Status : Outport  Port=6
  IL_Level_CAN_Data : Outport  Port=7
  IL_Level_CAN_Status : Outport  Port=8
  wires:
  rpIgnSubstate_IgnitionSubstate/1 -> rpIgnSubstate_IgnitionSubstate_out/1
  rpVehicleAppMode_WSSCurrentVehicleState/1 -> rpVehicleAppMode_WSSCurrentVehicleState_out/1
  rp_TFTDisplayOn_TFTDisplayOn/1 -> rp_TFTDisplayOn_TFTDisplayOn_out/1
  rp_StopPwmUpdate_channel_id/1 -> Terminator12/1
  rp_PowerTrain_State_PowerTrain_Flag/1 -> Terminator2/1
  rp_ClusterMode_WSSCurrentClusterMode/1 -> rp_ClusterMode_WSSCurrentClusterMode_out/1
  rp_Dcm_stop_app_AppId/1 -> Terminator3/1
  rpEtmSts_Illum_Status/1 -> Terminator4/1
  rpIllum_Etm_IllumStatus/1 -> Terminator5/1
  rp_custom_reset_CurrentUserID/1 -> Terminator6/1
  rp_custom_reset_CustomizeReset/1 -> Terminator7/1
  rp_custom_reset_SettingResetResult/1 -> Terminator8/1
  rpEtmTTSts_IllumStatus/1 -> Terminator9/1
  rp_Diag2F_Rheo_Diag_RheoStat/1 -> Terminator/1
  rp_EcoRunPresenceFlag_EcoRunPresenceFlag/1 -> Terminator1/1
  Constant/1 -> RxCan_GetSignalValue/1
  Constant1/1 -> RxCan_GetSignalValue1/1
  RxCan_GetSignalValue/1 -> IL_Mode_CAN_Data/1
  RxCan_GetSignalValue1/2 -> IL_Level_CAN_Status/1
  RxCan_GetSignalValue1/1 -> IL_Level_CAN_Data/1
  RxCan_GetSignalValue/2 -> IL_Mode_CAN_Status/1
  RxCan_GetSignalValue/3 -> Terminator10/1
  RxCan_GetSignalValue1/3 -> Terminator11/1
  rp_Ctrl_Ready_to_Sleep_Ready_to_Sleep/1 -> Terminator15/1
  rp_IlumDayNightStatus_Day_Night_Status/1 -> Terminator14/1
  rp_IlumDayNightRequired_IlumDayNightRequired/1 -> Terminator13/1

== system Mdl_Dim/Mdl_Dim_Task_sys/InputHarness/Simulation ==

== system Mdl_Dim/Mdl_Dim_Task_sys/OutputHarness/CodeGeneration ==
  pp_IllumCtrl_Ip_IllumCtrl_Ip_Data_in : Inport  OutDataTypeStr=Bus:IllumCtrl_Ip  PortDimensions=1
  pp_IllumCtrl_Ip_IllumCtrl_Ip_Data : Outport  OutDataTypeStr=Bus:IllumCtrl_Ip  PortDimensions=1
  wires:
  pp_IllumCtrl_Ip_IllumCtrl_Ip_Data_in/1 -> pp_IllumCtrl_Ip_IllumCtrl_Ip_Data/1

== system Mdl_Dim/Mdl_Dim_Task_sys/OutputHarness/Simulation ==
  pp_IlumDayNightRequired_ilumDNRequired : Outport  OutDataTypeStr=uint8  PortDimensions=1
  pp_IlumDayNightStatus_illumDNStatus : Outport  Port=2  OutDataTypeStr=uint8  PortDimensions=1
  pp_IlumStep_IllumStepValue : Outport  Port=3  OutDataTypeStr=uint8  PortDimensions=1
  pp_RGBStep_RGBStepValue : Outport  Port=4  OutDataTypeStr=uint16  PortDimensions=1
  pp_illumStarterstatus_StarterStatus_Out : Outport  Port=5  OutDataTypeStr=uint8  PortDimensions=1
  pp_illumRheostatOnSTimer_Rheostat_OnSTime : Outport  Port=6  OutDataTypeStr=uint16  PortDimensions=1
  pp_IlluminationDuty_DutyValue : Outport  Port=7  OutDataTypeStr=uint16  PortDimensions=1
  pp_RheoSwStatus_SwitchStatus : Outport  Port=8  OutDataTypeStr=uint8  PortDimensions=1
  pp_illum_rheostat_change_RheoUpdateVal : Outport  Port=9  OutDataTypeStr=uint8  PortDimensions=1
  pp_RheoSwRaw_Status_RawdataStatus : Outport  Port=10  OutDataTypeStr=uint8  PortDimensions=1
  pp_Illum_Transstep_Trans_Stepvlaue : Outport  Port=11  OutDataTypeStr=uint8  PortDimensions=1
  pp_RheostatDayStep_RheostatDayStep : Outport  Port=12  OutDataTypeStr=uint8  PortDimensions=1
  pp_RheostatNightStep_RheostatNightStep : Outport  Port=13  OutDataTypeStr=uint8  PortDimensions=1
  pp_RHUP_Dbc_RHUP_Dbc : Outport  Port=14  OutDataTypeStr=uint8  PortDimensions=1
  pp_RHDW_Dbc_RHDW_Dbc : Outport  Port=15  OutDataTypeStr=uint8  PortDimensions=1
  pp_RheostatSwType_RheostatSwType : Outport  Port=16  OutDataTypeStr=uint8  PortDimensions=1
  pp_RheostatONSStatus_RheostatONSStatus : Outport  Port=17  OutDataTypeStr=uint8  PortDimensions=1
  pp_IllumCtrl_Ip_IllumCtrl_Ip_Data : Outport  Port=18  OutDataTypeStr=Bus:IllumCtrl_Ip  PortDimensions=1

== system Mdl_Dim/Mdl_Dim_Task_sys/Subsystem/CANCommDet ==
  CANCommDet : TriggerPort  TriggerType=function-call  IsSimulinkFunction=on  FunctionName=CANCommDet  FunctionVisibility=scoped  VariantControl=(inherit)
  Compare To Constant : simulink/Logic and Bit Operations/Compare To Constant  relop===  const=RTE_E_MAX_AGE_EXCEEDED  OutDataTypeStr=boolean
  Compare To Constant1 : simulink/Logic and Bit Operations/Compare To Constant  relop===  const=RTE_E_NEVER_RECEIVED  OutDataTypeStr=boolean
  Constant : Constant  Value=CAN_COMUN_FAIL
  Constant1 : Constant  Value=CAN_COMUN_ACTIVE
  Constant2 : Constant  Value=CAN_COMUN_FAIL
  Switch : Switch  Criteria=u2 ~= 0  SaturateOnIntegerOverflow=off  InputSameDT=off
  Switch1 : Switch  Criteria=u2 ~= 0  SaturateOnIntegerOverflow=off  InputSameDT=off
  CAN_Status : ArgIn  DisableCoverage=on  OutDataTypeStr=uint8  ArgumentName=CAN_Status
  StatusDet : ArgOut  DisableCoverage=on  OutDataTypeStr=uint8  ArgumentName=StatusDet
  wires:
  Switch/1 -> StatusDet/1
  Constant2/1 -> Switch1/1
  Compare To Constant1/1 -> Switch1/2
  Compare To Constant/1 -> Switch/2
  Constant/1 -> Switch/1
  Constant1/1 -> Switch1/3
  Switch1/1 -> Switch/3
  CAN_Status/1 -> Compare To Constant1/1, Compare To Constant/1

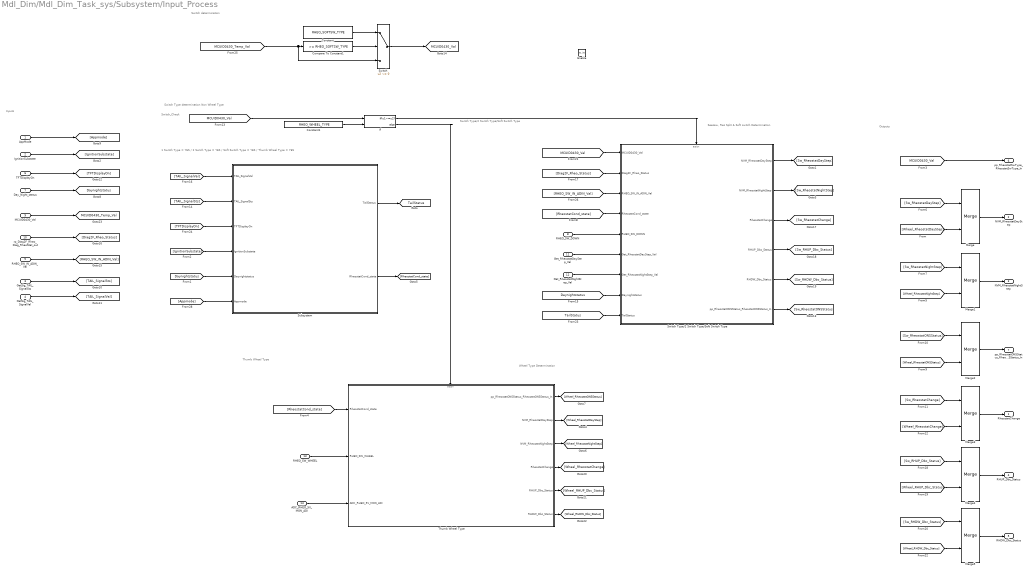
== system Mdl_Dim/Mdl_Dim_Task_sys/Subsystem/Input_Process ==
  note: Inputs
  note: Seesaw, Res Split & Soft switch Determination
  note: Switch determination
  note: Switch Type determination Non Wheel Type
  note: Switch_Check
  note: Outputs
  note: Thumb Wheel Type
  note: Switch Type/2 Switch Type/Soft Switch Type
  note: 1 Switch Type = YES / 2 Swtch Type = YES / Soft Switch Type = YES / Thumb Wheel Type = YES
  note: Wheel Type Determination
  AppMode : Inport
  IgnitionSubstate : Inport  Port=2
  GetSig_TAIL_SignalSts : Inport  Port=3
  GetSig_TAIL_SignalVal : Inport  Port=4
  RHEO_SW_IN_ADIN_Val : Inport  Port=5
  TFTDisplayOn : Inport  Port=6
  Day_Night_status : Inport  Port=7
  RHEO_SW_DOWN : Inport  Port=8
  MCUID0430_Val : Inport  Port=9
  rp_Diag2F_Rheo_Diag_RheoStat_out : Inport  Port=10
  Get_RheostatDayStep_Val : Inport  Port=11
  Get_RheostatNightStep_Val : Inport  Port=12
  RHEO_SW_WHEEL : Inport  Port=13
  ADC_RHEO_5V_MON_ADI : Inport  Port=14
  Enable : EnablePort
  Compare To Constant1 : simulink/Logic and Bit Operations/Compare To Constant  relop=>=  const=RHEO_SOFTSW_TYPE  OutDataTypeStr=boolean
  Constant : Constant  Value=RHEO_SOFTSW_TYPE
  Constant1 : Constant  Value=RHEO_WHEEL_TYPE  OutDataTypeStr=Inherit: Inherit via back propagation
  If : If  NumInputs=2  IfExpression=u1~=u2
  Merge{,1..5} (6 alike) : Merge
  Subsystem : Subsystem
  Switch : Switch  Criteria=u2 ~= 0  SaturateOnIntegerOverflow=off  InputSameDT=off
  Switch Type/2 Switch Type/Soft Switch Type : Subsystem  RTWFcnName=ONE_TWO_SOFT_SWITCH_HANDLING
      settings: RTWSystemCode=Nonreusable function  RTWFcnNameOpts=User specified  FunctionInterfaceSpec=Allow arguments (Optimized)
  Thumb Wheel Type : Subsystem  RTWFcnName=Thumb_Wheel_Type
      settings: RTWSystemCode=Nonreusable function  RTWFcnNameOpts=User specified  FunctionInterfaceSpec=Allow arguments (Optimized)
  RheostatChange : Outport  VectorParamsAs1DForOutWhenUnconnected=off
  "NVM_RheostatDayStep " : Outport  Port=2  VectorParamsAs1DForOutWhenUnconnected=off
  NVM_RheostatNightStep : Outport  Port=3  VectorParamsAs1DForOutWhenUnconnected=off
  RHUP_Dbc_Status : Outport  Port=4  VectorParamsAs1DForOutWhenUnconnected=off
  RHDW_Dbc_Status : Outport  Port=5  VectorParamsAs1DForOutWhenUnconnected=off
  pp_RheostatSwType_RheostatSwType_In : Outport  Port=6  VectorParamsAs1DForOutWhenUnconnected=off
  pp_RheostatONSStatus_RheostatONSStatus_In : Outport  Port=7  VectorParamsAs1DForOutWhenUnconnected=off
  tag scope: Daynightstatus=global, MCUID0430_Temp_Val=global, MCUID0430_Val=global, TailStatus=global
  wires:
  IgnitionSubstate/1 -> [IgnitionSubstate]
  AppMode/1 -> [Appmode]
  Day_Night_status/1 -> [Daynightstatus]
  RHEO_SW_IN_ADIN_Val/1 -> [RHEO_SW_IN_ADIN_Val]
  rp_Diag2F_Rheo_Diag_RheoStat_out/1 -> [Diag2F_Rheo_Status]
  GetSig_TAIL_SignalSts/1 -> [TAIL_SignalSts]
  GetSig_TAIL_SignalVal/1 -> [TAIL_SignalVal]
  Subsystem/1(TailStatus) -> [TailStatus]
  [TAIL_SignalVal] -> Subsystem/1(TAIL_SignalVal)
  [TAIL_SignalSts] -> Subsystem/2(TAIL_SignalSts)
  TFTDisplayOn/1 -> [TFTDisplayOn]
  [TFTDisplayOn] -> Subsystem/3(TFTDisplayOn)
  Subsystem/2(RheostatCond_state) -> [RheostatCond_state]
  [IgnitionSubstate] -> Subsystem/4(IgnitionSubstate)
  [Daynightstatus] -> Subsystem/5(Daynightstatus)
  RHEO_SW_DOWN/1 -> Switch Type/2 Switch Type/Soft Switch Type/5(RHEO_SW_DOWN)
  [MCUID0430_Val] -> Switch Type/2 Switch Type/Soft Switch Type/1(MCUID0430_Val)
  [Diag2F_Rheo_Status] -> Switch Type/2 Switch Type/Soft Switch Type/2(Diag2F_Rheo_Status)
  [RHEO_SW_IN_ADIN_Val] -> Switch Type/2 Switch Type/Soft Switch Type/3(RHEO_SW_IN_ADIN_Val)
  [RheostatCond_state] -> Switch Type/2 Switch Type/Soft Switch Type/4(RheostatCond_state)
  Get_RheostatDayStep_Val/1 -> Switch Type/2 Switch Type/Soft Switch Type/6(Get_RheostatDayStep_Val)
  Get_RheostatNightStep_Val/1 -> Switch Type/2 Switch Type/Soft Switch Type/7(Get_RheostatNightStep_Val)
  [Daynightstatus] -> Switch Type/2 Switch Type/Soft Switch Type/8(Daynightstatus)
  [MCUID0430_Val] -> pp_RheostatSwType_RheostatSwType_In/1
  ADC_RHEO_5V_MON_ADI/1 -> Thumb Wheel Type/3(ADC_RHEO_5V_MON_ADI)
  RHEO_SW_WHEEL/1 -> Thumb Wheel Type/2(RHEO_SW_WHEEL)
  [RheostatCond_state] -> Thumb Wheel Type/1(RheostatCond_state)
  Merge/1 -> "NVM_RheostatDayStep "/1
  Merge1/1 -> NVM_RheostatNightStep/1
  Switch Type/2 Switch Type/Soft Switch Type/1("NVM_RheostatDayStep ") -> [Sw_RheostatDayStep]
  Switch Type/2 Switch Type/Soft Switch Type/2(NVM_RheostatNightStep) -> [Sw_RheostatNightStep]
  Thumb Wheel Type/2("NVM_RheostatDayStep ") -> [Wheel_RheostatDayStep]
  Thumb Wheel Type/3(NVM_RheostatNightStep) -> [Wheel_RheostatNightStep]
  [Sw_RheostatDayStep] -> Merge/1
  [Wheel_RheostatDayStep] -> Merge/2
  [Wheel_RheostatNightStep] -> Merge1/2
  [Sw_RheostatNightStep] -> Merge1/1
  [Sw_RheostatONSStatus] -> Merge2/1
  [Wheel_RheostatONSStatus] -> Merge2/2
  Merge2/1 -> pp_RheostatONSStatus_RheostatONSStatus_In/1
  Thumb Wheel Type/1(pp_RheostatONSStatus_RheostatONSStatus_In) -> [Wheel_RheostatONSStatus]
  Switch Type/2 Switch Type/Soft Switch Type/6(pp_RheostatONSStatus_RheostatONSStatus_In) -> [Sw_RheostatONSStatus]
  [Wheel_RheostatChange] -> Merge3/2
  [Sw_RheostatChange] -> Merge3/1
  Merge3/1 -> RheostatChange/1
  [Sw_RHUP_Dbc_Status] -> Merge4/1
  [Wheel_RHUP_Dbc_Status] -> Merge4/2
  Merge4/1 -> RHUP_Dbc_Status/1
  [Sw_RHDW_Dbc_Status] -> Merge5/1
  [Wheel_RHDW_Dbc_Status] -> Merge5/2
  Merge5/1 -> RHDW_Dbc_Status/1
  Thumb Wheel Type/4(RheostatChange) -> [Wheel_RheostatChange]
  Thumb Wheel Type/5(RHUP_Dbc_Status) -> [Wheel_RHUP_Dbc_Status]
  Thumb Wheel Type/6(RHDW_Dbc_Status) -> [Wheel_RHDW_Dbc_Status]
  Switch Type/2 Switch Type/Soft Switch Type/3(RheostatChange) -> [Sw_RheostatChange]
  Switch Type/2 Switch Type/Soft Switch Type/4(RHUP_Dbc_Status) -> [Sw_RHUP_Dbc_Status]
  Switch Type/2 Switch Type/Soft Switch Type/5(RHDW_Dbc_Status) -> [Sw_RHDW_Dbc_Status]
  [MCUID0430_Temp_Val] -> Switch/3, Compare To Constant1/1
  Compare To Constant1/1 -> Switch/2
  Constant/1 -> Switch/1
  Switch/1 -> [MCUID0430_Val]
  MCUID0430_Val/1 -> [MCUID0430_Temp_Val]
  [Appmode] -> Subsystem/6(Appmode)
  [TailStatus] -> Switch Type/2 Switch Type/Soft Switch Type/9(TailStatus)
  [MCUID0430_Val] -> If/1
  If/1 -> Switch Type/2 Switch Type/Soft Switch Type/Action
  If/2 -> Thumb Wheel Type/Action
  Constant1/1 -> If/2

== system Mdl_Dim/Mdl_Dim_Task_sys/Subsystem/Subsystem2 ==
  Enable : EnablePort
  Compare To Constant : simulink/Logic and Bit Operations/Compare To Constant  relop=>  const=1  OutDataTypeStr=boolean
  Compare To Constant1 : simulink/Logic and Bit Operations/Compare To Constant  relop=>  const=4  OutDataTypeStr=boolean
  Compare To Constant2 : simulink/Logic and Bit Operations/Compare To Constant  relop=>  const=21  OutDataTypeStr=uint8
  Constant : Constant  OutDataTypeStr=uint8
  Constant1 : Constant  OutDataTypeStr=uint8
  Constant2 : Constant  OutDataTypeStr=uint8
  Constant3 : Constant  Value=10  OutDataTypeStr=uint8
  Constant4 : Constant  Value=INDEX_MCUID0340
  Constant7 : Constant  Value=INDEX_MCUID0341
  Constant8 : Constant  Value=INDEX_MCUID0430
  Data Store Write : DataStoreWrite  DataStoreName=l_dimming_Init_MCU  IndexOptions=Index vector (dialog)  Indices=1  OutputSizes=1
  Data Store Write1 : DataStoreWrite  DataStoreName=l_Prev_NVM_RheostatDayStep  IndexOptions=Index vector (dialog)  Indices=1  OutputSizes=1
  Data Store Write2 : DataStoreWrite  DataStoreName=l_Prev_NVM_RheostatNightStep  IndexOptions=Index vector (dialog)  Indices=1  OutputSizes=1
  Data Store Write3 : DataStoreWrite  DataStoreName=l_Dim_MCUID0340_val  IndexOptions=Index vector (dialog)  Indices=1  OutputSizes=1
  Data Store Write4 : DataStoreWrite  DataStoreName=MCUID0341  IndexOptions=Index vector (dialog)  Indices=1  OutputSizes=1
  Dimming_MCU_ID : FunctionCaller  FunctionPrototype=pMCUCONST_Data_dim_430_341 = Rte_Call_rp_CS_MCUConst_Mdl_dimming_Mdl_dimming_MCUID()  InputArgumentSpecifications=<Enter example>  OutputArgumentSpecifications=uint8(zeros(1,3))
  NVM_Adapter_GetNVM_RheostatDayStep : FunctionCaller  FunctionPrototype=pNvmData = NVM_Adapter_GetNVM_RheostatDayStep()  InputArgumentSpecifications=<Enter example>  OutputArgumentSpecifications=uint8(1)
  NVM_Adapter_GetNVM_RheostatNightStep : FunctionCaller  FunctionPrototype=pNvmData = NVM_Adapter_GetNVM_RheostatNightStep()  InputArgumentSpecifications=<Enter example>  OutputArgumentSpecifications=uint8(1)
  Selector1 : Selector  IndexMode=Zero-based  InputPortWidth=3  IndexOptions=Index vector (port)  Indices=[1 3]  OutputSizes=1
  Selector2 : Selector  IndexMode=Zero-based  InputPortWidth=3  IndexOptions=Index vector (port)  Indices=[1 3]  OutputSizes=1
  Selector3 : Selector  IndexMode=Zero-based  InputPortWidth=3  IndexOptions=Index vector (port)  Indices=[1 3]  OutputSizes=1
  Switch : Switch  Criteria=u2 ~= 0  SaturateOnIntegerOverflow=off  InputSameDT=off
  Switch1 : Switch  Criteria=u2 ~= 0  SaturateOnIntegerOverflow=off  InputSameDT=off
  Switch3 : Switch  Criteria=u2 ~= 0  SaturateOnIntegerOverflow=off  InputSameDT=off
  MCUID0430_Val : Outport  VectorParamsAs1DForOutWhenUnconnected=off
  wires:
  Constant8/1 -> Selector3/2
  Constant7/1 -> Selector2/2
  Selector3/1 -> Switch1/3, Compare To Constant1/1
  Dimming_MCU_ID/1 -> Selector1/1, Selector3/1, Selector2/1  "fl_Max_value"
  Compare To Constant/1 -> Switch/2
  Switch/1 -> Data Store Write4/1
  Selector2/1 -> Switch/3, Compare To Constant/1
  Constant/1 -> Switch/1
  Switch1/1 -> MCUID0430_Val/1
  Compare To Constant1/1 -> Switch1/2
  Constant1/1 -> Switch1/1
  Constant2/1 -> Data Store Write/1
  NVM_Adapter_GetNVM_RheostatNightStep/1 -> Data Store Write2/1
  NVM_Adapter_GetNVM_RheostatDayStep/1 -> Data Store Write1/1
  Constant4/1 -> Selector1/2
  Constant3/1 -> Switch3/1
  Compare To Constant2/1 -> Switch3/2
  Selector1/1 -> Switch3/3, Compare To Constant2/1
  Switch3/1 -> Data Store Write3/1

== system Mdl_Dim/Mdl_Dim_Task_sys/Subsystem/Input_Process/Subsystem ==
  note: Tail Status Determination
  note: Rheo Condition Determination
  TAIL_SignalVal : Inport
  TAIL_SignalSts : Inport  Port=2
  TFTDisplayOn : Inport  Port=3
  IgnitionSubstate : Inport  Port=4
  Daynightstatus : Inport  Port=5
  Appmode : Inport  Port=6
  Function Caller3 : FunctionCaller  FunctionPrototype=StatusDet = CANCommDet(CAN_Status)  InputArgumentSpecifications=<Enter example>  OutputArgumentSpecifications=<Enter example>
  Rheostat_Control_Enable_Condition_Determination : Truth Table  TreatAsAtomicUnit=on
      settings: RTWSystemCode=Nonreusable function  RTWFcnNameOpts=Use subsystem name  FunctionInterfaceSpec=Allow arguments (Optimized)
  TAIL_Status_Processing : Truth Table  TreatAsAtomicUnit=on
      settings: RTWSystemCode=Nonreusable function  RTWFcnNameOpts=Use subsystem name  FunctionInterfaceSpec=Allow arguments (Optimized)
  Unit Delay1 : UnitDelay  SampleTime=-1  StateName=l_Prev_Tailstatus_Status  HasFrameUpgradeWarning=on
  TailStatus : Outport  VectorParamsAs1DForOutWhenUnconnected=off
  RheostatCond_state : Outport  Port=2  VectorParamsAs1DForOutWhenUnconnected=off
  wires:
  Appmode/1 -> TAIL_Status_Processing/4(Appmode)
  Unit Delay1/1 -> TAIL_Status_Processing/5(PrevTailStsVal)
  TAIL_Status_Processing/1(TailStatus) -> Unit Delay1/1, [TailStatus], TailStatus/1  "TailStatus"
  Function Caller3/1 -> TAIL_Status_Processing/2(TailCANstatus)
  [IgnitionSubstate] -> TAIL_Status_Processing/1(Ignitionmode)
  TAIL_SignalVal/1 -> TAIL_Status_Processing/3(TailCanVal)
  TAIL_SignalSts/1 -> Function Caller3/1
  Rheostat_Control_Enable_Condition_Determination/1(RheostatCond_state) -> RheostatCond_state/1
  TFTDisplayOn/1 -> Rheostat_Control_Enable_Condition_Determination/1(TFTDisplayOn)
  [TailStatus] -> Rheostat_Control_Enable_Condition_Determination/3(TailStatus_Val)
  Daynightstatus/1 -> Rheostat_Control_Enable_Condition_Determination/4(IlumDayNightStatus)
  IgnitionSubstate/1 -> [IgnitionSubstate]
  [IgnitionSubstate] -> Rheostat_Control_Enable_Condition_Determination/2(Ignstatus)
